simulink model "Sim_exercise32"  (R2014b)
settings: Solver=VariableStepAuto  StartTime=0.0  StopTime=0.1  RelTol=1e-3
values from neighbouring files (symbols this model uses):
  Amplitude = 2    [Exercise_3.m]
  dm = 3.8E-6    (= 3.8e-06)    [Exercise_1.m]    (also in Exercise_3.m)
  Freq = 2    [Exercise_3.m]
  Jeq = Jm + (J1+J2)/(n^2)    (= 2.186e-06)    [Exercise_1.m]    (also in Exercise_3.m)
  Kemf = 137*2*pi/60    (= 14.3466064514)    [Exercise_1.m]    (also in Exercise_3.m = 0.0697028947848)
  Km = 69.7E-3    (= 0.0697)    [Exercise_1.m]    (also in Exercise_3.m)
  n = 5    [Exercise_1.m]    (also in Exercise_3.m)
  R = 112    [Exercise_1.m]    (also in Exercise_3.m)
  Sine_wave = 1    [Exercise_3.m]
  Tc = 1E-3    (= 0.001)    [Exercise_3.m]
  voltage = 1    [Exercise_3.m]
libraries: simulink x1
settings Model: Creator=sofianh  LastModifiedBy=sofianh
settings DataIOCC: SaveFormat=Dataset
settings OptimizationCC: UseDivisionForNetSlopeComputation=off  SimCompilerOptimization=off
settings DebuggingCC: SolverPrmCheckMsg=none  FrameProcessingCompatibilityMsg=error  AllowSymbolicDim=off
settings HardwareCC: ProdBitPerPointer=64  ProdLargestAtomicFloat=Float  ProdIntDivRoundTo=Zero  ProdEndianess=LittleEndian  ProdWordSize=64  ProdHWDeviceType=Intel->x86-64 (Windows64)
settings RTWCC: RTWCompilerOptimization=off
settings GRTTargetCC: GeneratePreprocessorConditionals=Use local settings
settings ConfigComp: CovMetricSettings=dw  CovHtmlReporting=on  CovSaveCumulativeToWorkspaceVar=on  CovSaveSingleToWorkspaceVar=on  CovExternalEMLEnable=off

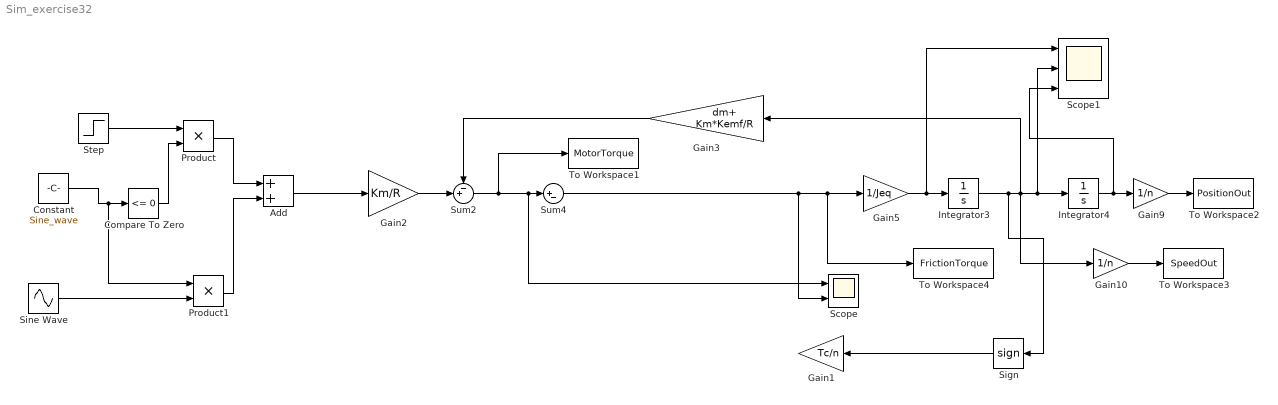
== system Sim_exercise32 ==
  Add : Sum
  Compare To Zero : simulink/Logic and Bit Operations/Compare To Zero  relop=<=  OutDataTypeStr=boolean
  Constant : Constant  Value=Sine_wave
  Gain1 : Gain  Gain=Tc/n
  Gain10 : Gain  Gain=1/n
  Gain2 : Gain  Gain=Km/R
  Gain3 : Gain  Gain=dm+ Km*Kemf/R
  Gain5 : Gain  Gain=1/Jeq
  Gain9 : Gain  Gain=1/n
  Integrator3 : Integrator
  Integrator4 : Integrator
  Product : Product
  Product1 : Product
  Scope : Scope  NumInputPorts=2
      settings: YMin=0.00052~-5  YMax=0.00072~5
  Scope1 : Scope  NumInputPorts=3
      settings: YMin=-100~-1e-05~-5e-07  YMax=200~9e-05~2.5e-06
  Sign : Signum  ZeroCross=off
  Sine Wave : Sin  Amplitude=Amplitude  Frequency=Freq  SampleTime=0
  Step : Step  Time=0  After=voltage  SampleTime=0
  Sum2 : Sum  Inputs=-+|
  Sum4 : Sum  Inputs=|+-
  To Workspace1 : ToWorkspace  VariableName=MotorTorque  SaveFormat=Structure With Time  SampleTime=-1
  To Workspace2 : ToWorkspace  VariableName=PositionOut  SaveFormat=Structure With Time  SampleTime=-1
  To Workspace3 : ToWorkspace  VariableName=SpeedOut  SaveFormat=Structure With Time  SampleTime=-1
  To Workspace4 : ToWorkspace  VariableName=FrictionTorque  SaveFormat=Structure With Time  SampleTime=-1
  wires:
  Gain2/1 -> Sum2/2
  Integrator3/1 -> Sign/1, Scope1/2, Integrator4/1, Gain10/1, Gain3/1
  Gain3/1 -> Sum2/1
  Sum4/1 -> To Workspace4/1, Gain5/1, Scope/2
  Gain5/1 -> Scope1/1, Integrator3/1
  Integrator4/1 -> Scope1/3, Gain9/1
  Gain9/1 -> To Workspace2/1
  Gain10/1 -> To Workspace3/1
  Add/1 -> Gain2/1
  Sum2/1 -> To Workspace1/1, Sum4/1, Scope/1
  Sign/1 -> Gain1/1
  Step/1 -> Product/1
  Constant/1 -> Product1/1, Compare To Zero/1
  Sine Wave/1 -> Product1/2
  Product/1 -> Add/1
  Product1/1 -> Add/2
  Compare To Zero/1 -> Product/2
